simulink model "ultra"  (R2020b)
settings: Solver=FixedStepDiscrete  StartTime=0.0  StopTime=10.0  FixedStep=0.0005  RelTol=1e-3  EnableMultiTasking=on
undefined symbols (not defined in the file): acc_calmax1, acc_calmax2, acc_calmin1, acc_calmin2, akemancanshu, bre, bre_calmax, bre_calmin, ecucoder_acal, I_AN01_5K1, I_AN03_5V, I_AN04_5V, kd, ki, kp, leftmax, O_SW06_HS1A, rightmax, T_add, T_del, tiaoshi, zhiling
libraries: ec5744lib x215, canmsglib x75, simulink x10
(part 4 of 7)

== system ultra/RX/284 286右前/Subsystem2/Subsystem ==
  ID : Inport
  msg : Inport  Port=2
  Enable : EnablePort
  CAN Pack : canmsglib/CAN Pack  Commented=on  CANdbFile=D:\desktop\enable.dbc  MsgList=(none)  MsgName=AMK_ActualValue1  MsgIDType=Standard (11-bit identifier)  MsgIdentifier=643  MsgLength=8  Remote=off  ApplyMinMax=off  BusOutput=off  SignalInfo={'AMK_ActualVelocity','16','16','LE','signed','Standard','0','1','0','0','65535';'AMK_MagnetizingCurrent','48','16','LE','signed','Standard','0','1','0','0','65535';'AMK_TorqueCurrent','32','16','LE','signed','Standard','0','1','0','0','65535';'AMK_bDcOn1','12','1','LE','unsigned','Standard','0','1','0','0','1';'AMK_bDerating1','15','1','LE','unsigned','Standard','0','1','0','0','1';'AMK_bError1','9','1','LE','unsigned','Standard','0','1','0','0','1';'AMK_bInverterOn1','14','1','LE','unsigned','Standard','0','1','0','0','1';'AMK_bQuitDcOn1','11','1','LE','unsigned','Standard','0','1','0','0','1';'AMK_bQuitInverterOn1','13','1','LE','unsigned','Standard','0','1','0','0','1';'AMK_bReserve1','0','8','LE','unsigned','Standard','0','1','0','0','255';'AMK_bSystemReady1','8','1','LE','unsigned','Standard','0','1','0','0','1';'AMK_bWarn1','10','1','LE','unsigned','Standard','0','1','0','0','1'}
      settings: SourceProductBaseCode=ME,XP,VN  DataFormat=CANdb specified signals
  CAN Unpack : canmsglib/CAN Unpack  CANdbFile=D:\desktop\刘科良\HRT23赛季刘科良\CANdbc\enable - youqian.dbc  MsgList=(none)  MsgName=AMK_ActualValue1  MsgIDType=Standard (11-bit identifier)  MsgIdentifier=644  MsgLength=8  SignalInfo={'AMK_ActualVelocity','16','16','LE','signed','Standard','0','1','0','0','65535';'AMK_MagnetizingCurrent','48','16','LE','signed','Standard','0','1','0','0','65535';'AMK_TorqueCurrent','32','16','LE','signed','Standard','0','1','0','0','65535';'AMK_bDcOn1','12','1','LE','unsigned','Standard','0','1','0','0','1';'AMK_bDerating1','15','1','LE','unsigned','Standard','0','1','0','0','1';'AMK_bError1','9','1','LE','unsigned','Standard','0','1','0','0','1';'AMK_bInverterOn1','14','1','LE','unsigned','Standard','0','1','0','0','1';'AMK_bQuitDcOn1','11','1','LE','unsigned','Standard','0','1','0','0','1';'AMK_bQuitInverterOn1','13','1','LE','unsigned','Standard','0','1','0','0','1';'AMK_bReserve1','0','8','LE','unsigned','Standard','0','1','0','0','255';'AMK_bSystemReady1','8','1','LE','unsigned','Standard','0','1','0','0','1';'AMK_bWarn1','10','1','LE','unsigned','Standard','0','1','0','0','1'}  IDPort=off  TimestampPort=off  ErrorPort=off  RemotePort=off  LengthPort=off  StatusPort=off  ApplyMinMax=off
      settings: SourceProductBaseCode=ME,XP,VN  DataFormat=CANdb specified signals
  CANPackMessage : ec5744lib/RapidECU_U4B/04CANCommunication/CANPackMessage  Commented=on  datalength=8  sampletime=-1
      settings: SourceProductName=ECUCoder for MPC5744
  CANUnPackMessage : ec5744lib/RapidECU_U4B/04CANCommunication/CANUnPackMessage  datalength=8  canmessagetype=Standard(11-bit ID)  sampletime=-1
      settings: SourceProductName=ECUCoder for MPC5744
  Data Store Write : DataStoreWrite  DataStoreName=dianji_velcoity_youqian
  Data Store Write1 : DataStoreWrite  DataStoreName=dianji_velcoity_youqian1
  MATLAB Function : MATLAB Function  TreatAsAtomicUnit=on
  wires:
  msg/1 -> CANUnPackMessage/2
  CANUnPackMessage/1 -> CAN Unpack/1
  ID/1 -> CANUnPackMessage/1
  CANPackMessage/1 -> ?
  CAN Pack/1 -> CANPackMessage/1
  CAN Unpack/1 -> Data Store Write1/1, MATLAB Function/1(u)
  MATLAB Function/1(y) -> Data Store Write/1

== system ultra/RX/287 289右后/Subsystem1/Subsystem ==
  ID : Inport
  msg : Inport  Port=2
  Enable : EnablePort
  CAN Pack : canmsglib/CAN Pack  Commented=on  CANdbFile=D:\desktop\enable.dbc  MsgList=(none)  MsgName=AMK_ActualValue1  MsgIDType=Standard (11-bit identifier)  MsgIdentifier=643  MsgLength=8  Remote=off  ApplyMinMax=off  BusOutput=off  SignalInfo={'AMK_ActualVelocity','16','16','LE','signed','Standard','0','1','0','0','65535';'AMK_MagnetizingCurrent','48','16','LE','signed','Standard','0','1','0','0','65535';'AMK_TorqueCurrent','32','16','LE','signed','Standard','0','1','0','0','65535';'AMK_bDcOn1','12','1','LE','unsigned','Standard','0','1','0','0','1';'AMK_bDerating1','15','1','LE','unsigned','Standard','0','1','0','0','1';'AMK_bError1','9','1','LE','unsigned','Standard','0','1','0','0','1';'AMK_bInverterOn1','14','1','LE','unsigned','Standard','0','1','0','0','1';'AMK_bQuitDcOn1','11','1','LE','unsigned','Standard','0','1','0','0','1';'AMK_bQuitInverterOn1','13','1','LE','unsigned','Standard','0','1','0','0','1';'AMK_bReserve1','0','8','LE','unsigned','Standard','0','1','0','0','255';'AMK_bSystemReady1','8','1','LE','unsigned','Standard','0','1','0','0','1';'AMK_bWarn1','10','1','LE','unsigned','Standard','0','1','0','0','1'}
      settings: SourceProductBaseCode=ME,XP,VN  DataFormat=CANdb specified signals
  CAN Unpack : canmsglib/CAN Unpack  CANdbFile=D:\desktop\刘科良\HRT23赛季刘科良\CANdbc\enable - zuohou - 副本.dbc  MsgList=(none)  MsgName=AMK_ActualValue2  MsgIDType=Standard (11-bit identifier)  MsgIdentifier=649  MsgLength=8  SignalInfo={'AMK_ErrorInfo','32','16','LE','unsigned','Standard','0','1','0','0','65535';'AMK_TempIGBT','48','16','LE','signed','Standard','0','1','0','0','65535';'AMK_TempInverter','16','16','LE','signed','Standard','0','1','0','-32768','32767';'AMK_TempMotor','0','16','LE','signed','Standard','0','1','0','0','65535'}  IDPort=off  TimestampPort=off  ErrorPort=off  RemotePort=off  LengthPort=off  StatusPort=off  ApplyMinMax=off
      settings: SourceProductBaseCode=ME,XP,VN  DataFormat=CANdb specified signals
  CANPackMessage : ec5744lib/RapidECU_U4B/04CANCommunication/CANPackMessage  Commented=on  datalength=8  sampletime=-1
      settings: SourceProductName=ECUCoder for MPC5744
  CANUnPackMessage : ec5744lib/RapidECU_U4B/04CANCommunication/CANUnPackMessage  datalength=8  canmessagetype=Standard(11-bit ID)  sampletime=-1
      settings: SourceProductName=ECUCoder for MPC5744
  wires:
  msg/1 -> CANUnPackMessage/2
  CANUnPackMessage/1 -> CAN Unpack/1
  ID/1 -> CANUnPackMessage/1
  CANPackMessage/1 -> ?
  CAN Pack/1 -> CANPackMessage/1

== system ultra/RX/287 289右后/Subsystem2/Subsystem ==
  ID : Inport
  msg : Inport  Port=2
  Enable : EnablePort
  CAN Pack : canmsglib/CAN Pack  Commented=on  CANdbFile=D:\desktop\enable.dbc  MsgList=(none)  MsgName=AMK_ActualValue1  MsgIDType=Standard (11-bit identifier)  MsgIdentifier=643  MsgLength=8  Remote=off  ApplyMinMax=off  BusOutput=off  SignalInfo={'AMK_ActualVelocity','16','16','LE','signed','Standard','0','1','0','0','65535';'AMK_MagnetizingCurrent','48','16','LE','signed','Standard','0','1','0','0','65535';'AMK_TorqueCurrent','32','16','LE','signed','Standard','0','1','0','0','65535';'AMK_bDcOn1','12','1','LE','unsigned','Standard','0','1','0','0','1';'AMK_bDerating1','15','1','LE','unsigned','Standard','0','1','0','0','1';'AMK_bError1','9','1','LE','unsigned','Standard','0','1','0','0','1';'AMK_bInverterOn1','14','1','LE','unsigned','Standard','0','1','0','0','1';'AMK_bQuitDcOn1','11','1','LE','unsigned','Standard','0','1','0','0','1';'AMK_bQuitInverterOn1','13','1','LE','unsigned','Standard','0','1','0','0','1';'AMK_bReserve1','0','8','LE','unsigned','Standard','0','1','0','0','255';'AMK_bSystemReady1','8','1','LE','unsigned','Standard','0','1','0','0','1';'AMK_bWarn1','10','1','LE','unsigned','Standard','0','1','0','0','1'}
      settings: SourceProductBaseCode=ME,XP,VN  DataFormat=CANdb specified signals
  CAN Unpack : canmsglib/CAN Unpack  CANdbFile=C:\Users\Liu keliang\Desktop\HRT2023\HRT23赛季刘科良\CANdbc\enable - zuohou - 副本.dbc  MsgList=(none)  MsgName=AMK_ActualValue1  MsgIDType=Standard (11-bit identifier)  MsgIdentifier=647  MsgLength=8  SignalInfo={'AMK_ActualVelocity','16','16','LE','signed','Standard','0','1','0','0','65535';'AMK_MagnetizingCurrent','48','16','LE','signed','Standard','0','1','0','0','65535';'AMK_TorqueCurrent','32','16','LE','signed','Standard','0','1','0','0','65535';'AMK_bDcOn1','12','1','LE','unsigned','Standard','0','1','0','0','1';'AMK_bDerating1','15','1','LE','unsigned','Standard','0','1','0','0','1';'AMK_bError1','9','1','LE','unsigned','Standard','0','1','0','0','1';'AMK_bInverterOn1','14','1','LE','unsigned','Standard','0','1','0','0','1';'AMK_bQuitDcOn1','11','1','LE','unsigned','Standard','0','1','0','0','1';'AMK_bQuitInverterOn1','13','1','LE','unsigned','Standard','0','1','0','0','1';'AMK_bReserve1','0','8','LE','unsigned','Standard','0','1','0','0','255';'AMK_bSystemReady1','8','1','LE','unsigned','Standard','0','1','0','0','1';'AMK_bWarn1','10','1','LE','unsigned','Standard','0','1','0','0','1'}  IDPort=off  TimestampPort=off  ErrorPort=off  RemotePort=off  LengthPort=off  StatusPort=off  ApplyMinMax=off
      settings: SourceProductBaseCode=ME,XP,VN  DataFormat=CANdb specified signals
  CANPackMessage : ec5744lib/RapidECU_U4B/04CANCommunication/CANPackMessage  Commented=on  datalength=8  sampletime=-1
      settings: SourceProductName=ECUCoder for MPC5744
  CANUnPackMessage : ec5744lib/RapidECU_U4B/04CANCommunication/CANUnPackMessage  datalength=8  canmessagetype=Standard(11-bit ID)  sampletime=-1
      settings: SourceProductName=ECUCoder for MPC5744
  Data Store Write : DataStoreWrite  DataStoreName=dianji_velcoity_zuohou
  MATLAB Function : MATLAB Function  TreatAsAtomicUnit=on
  wires:
  msg/1 -> CANUnPackMessage/2
  CANUnPackMessage/1 -> CAN Unpack/1
  ID/1 -> CANUnPackMessage/1
  CANPackMessage/1 -> ?
  CAN Pack/1 -> CANPackMessage/1
  CAN Unpack/1 -> MATLAB Function/1(u)
  MATLAB Function/1(y) -> Data Store Write/1

== system ultra/RX/287 289右后/Subsystem3/Subsystem ==
  ID : Inport
  msg : Inport  Port=2
  Enable : EnablePort
  CAN Pack : canmsglib/CAN Pack  Commented=on  CANdbFile=D:\desktop\enable.dbc  MsgList=(none)  MsgName=AMK_ActualValue1  MsgIDType=Standard (11-bit identifier)  MsgIdentifier=643  MsgLength=8  Remote=off  ApplyMinMax=off  BusOutput=off  SignalInfo={'AMK_ActualVelocity','16','16','LE','signed','Standard','0','1','0','0','65535';'AMK_MagnetizingCurrent','48','16','LE','signed','Standard','0','1','0','0','65535';'AMK_TorqueCurrent','32','16','LE','signed','Standard','0','1','0','0','65535';'AMK_bDcOn1','12','1','LE','unsigned','Standard','0','1','0','0','1';'AMK_bDerating1','15','1','LE','unsigned','Standard','0','1','0','0','1';'AMK_bError1','9','1','LE','unsigned','Standard','0','1','0','0','1';'AMK_bInverterOn1','14','1','LE','unsigned','Standard','0','1','0','0','1';'AMK_bQuitDcOn1','11','1','LE','unsigned','Standard','0','1','0','0','1';'AMK_bQuitInverterOn1','13','1','LE','unsigned','Standard','0','1','0','0','1';'AMK_bReserve1','0','8','LE','unsigned','Standard','0','1','0','0','255';'AMK_bSystemReady1','8','1','LE','unsigned','Standard','0','1','0','0','1';'AMK_bWarn1','10','1','LE','unsigned','Standard','0','1','0','0','1'}
      settings: SourceProductBaseCode=ME,XP,VN  DataFormat=CANdb specified signals
  CAN Unpack : canmsglib/CAN Unpack  CANdbFile=C:\Users\Liu keliang\Desktop\HRT2023\HRT23赛季刘科良\CANdbc\enable - 副本.dbc  MsgList=AMK_ActualValue1  MsgName=AMK_ActualValue1  MsgIDType=Standard (11-bit identifier)  MsgIdentifier=647  MsgLength=8  SignalInfo={'AMK_ActualVelocity','16','16','LE','signed','Standard','0','1','0','0','65535';'AMK_MagnetizingCurrent','48','16','LE','signed','Standard','0','1','0','0','65535';'AMK_TorqueCurrent','32','16','LE','signed','Standard','0','1','0','0','65535';'AMK_bDcOn1','12','1','LE','unsigned','Standard','0','1','0','0','1';'AMK_bDerating1','15','1','LE','unsigned','Standard','0','1','0','0','1';'AMK_bError1','9','1','LE','unsigned','Standard','0','1','0','0','1';'AMK_bInverterOn1','14','1','LE','unsigned','Standard','0','1','0','0','1';'AMK_bQuitDcOn1','11','1','LE','unsigned','Standard','0','1','0','0','1';'AMK_bQuitInverterOn1','13','1','LE','unsigned','Standard','0','1','0','0','1';'AMK_bReserve1','0','8','LE','unsigned','Standard','0','1','0','0','255';'AMK_bSystemReady1','8','1','LE','unsigned','Standard','0','1','0','0','1';'AMK_bWarn1','10','1','LE','unsigned','Standard','0','1','0','0','1'}  IDPort=off  TimestampPort=off  ErrorPort=off  RemotePort=off  LengthPort=off  StatusPort=off  ApplyMinMax=off
      settings: SourceProductBaseCode=ME,XP,VN  DataFormat=CANdb specified signals
  CANPackMessage : ec5744lib/RapidECU_U4B/04CANCommunication/CANPackMessage  Commented=on  datalength=8  sampletime=-1
      settings: SourceProductName=ECUCoder for MPC5744
  CANUnPackMessage : ec5744lib/RapidECU_U4B/04CANCommunication/CANUnPackMessage  datalength=8  canmessagetype=Standard(11-bit ID)  sampletime=-1
      settings: SourceProductName=ECUCoder for MPC5744
  Data Store Write : DataStoreWrite  DataStoreName=dianji_velcoity_youhou
  Data Store Write1 : DataStoreWrite  DataStoreName=dianji_velcoity_youhou1
  MATLAB Function : MATLAB Function  TreatAsAtomicUnit=on
  wires:
  msg/1 -> CANUnPackMessage/2
  CANUnPackMessage/1 -> CAN Unpack/1
  ID/1 -> CANUnPackMessage/1
  CANPackMessage/1 -> ?
  CAN Pack/1 -> CANPackMessage/1
  MATLAB Function/1(y) -> Data Store Write/1
  CAN Unpack/1 -> Data Store Write1/1, MATLAB Function/1(u)

== system ultra/RX/288 290左后/Subsystem1/Subsystem ==
  ID : Inport
  msg : Inport  Port=2
  Enable : EnablePort
  CAN Pack : canmsglib/CAN Pack  Commented=on  CANdbFile=D:\desktop\enable.dbc  MsgList=(none)  MsgName=AMK_ActualValue1  MsgIDType=Standard (11-bit identifier)  MsgIdentifier=643  MsgLength=8  Remote=off  ApplyMinMax=off  BusOutput=off  SignalInfo={'AMK_ActualVelocity','16','16','LE','signed','Standard','0','1','0','0','65535';'AMK_MagnetizingCurrent','48','16','LE','signed','Standard','0','1','0','0','65535';'AMK_TorqueCurrent','32','16','LE','signed','Standard','0','1','0','0','65535';'AMK_bDcOn1','12','1','LE','unsigned','Standard','0','1','0','0','1';'AMK_bDerating1','15','1','LE','unsigned','Standard','0','1','0','0','1';'AMK_bError1','9','1','LE','unsigned','Standard','0','1','0','0','1';'AMK_bInverterOn1','14','1','LE','unsigned','Standard','0','1','0','0','1';'AMK_bQuitDcOn1','11','1','LE','unsigned','Standard','0','1','0','0','1';'AMK_bQuitInverterOn1','13','1','LE','unsigned','Standard','0','1','0','0','1';'AMK_bReserve1','0','8','LE','unsigned','Standard','0','1','0','0','255';'AMK_bSystemReady1','8','1','LE','unsigned','Standard','0','1','0','0','1';'AMK_bWarn1','10','1','LE','unsigned','Standard','0','1','0','0','1'}
      settings: SourceProductBaseCode=ME,XP,VN  DataFormat=CANdb specified signals
  CAN Unpack : canmsglib/CAN Unpack  CANdbFile=D:\desktop\刘科良\HRT23赛季刘科良\CANdbc\enable - youhou -.dbc  MsgList=(none)  MsgName=AMK_ActualValue2  MsgIDType=Standard (11-bit identifier)  MsgIdentifier=656  MsgLength=8  SignalInfo={'AMK_ErrorInfo','32','16','LE','unsigned','Standard','0','1','0','0','65535';'AMK_TempIGBT','48','16','LE','signed','Standard','0','1','0','0','65535';'AMK_TempInverter','16','16','LE','signed','Standard','0','1','0','-32768','32767';'AMK_TempMotor','0','16','LE','signed','Standard','0','1','0','0','65535'}  IDPort=off  TimestampPort=off  ErrorPort=off  RemotePort=off  LengthPort=off  StatusPort=off  ApplyMinMax=off
      settings: SourceProductBaseCode=ME,XP,VN  DataFormat=CANdb specified signals
  CANPackMessage : ec5744lib/RapidECU_U4B/04CANCommunication/CANPackMessage  Commented=on  datalength=8  sampletime=-1
      settings: SourceProductName=ECUCoder for MPC5744
  CANUnPackMessage : ec5744lib/RapidECU_U4B/04CANCommunication/CANUnPackMessage  datalength=8  canmessagetype=Standard(11-bit ID)  sampletime=-1
      settings: SourceProductName=ECUCoder for MPC5744
  wires:
  msg/1 -> CANUnPackMessage/2
  CANUnPackMessage/1 -> CAN Unpack/1
  ID/1 -> CANUnPackMessage/1
  CANPackMessage/1 -> ?
  CAN Pack/1 -> CANPackMessage/1

== system ultra/RX/288 290左后/Subsystem2/Subsystem ==
  ID : Inport
  msg : Inport  Port=2
  Enable : EnablePort
  CAN Pack : canmsglib/CAN Pack  Commented=on  CANdbFile=D:\desktop\enable.dbc  MsgList=(none)  MsgName=AMK_ActualValue1  MsgIDType=Standard (11-bit identifier)  MsgIdentifier=643  MsgLength=8  Remote=off  ApplyMinMax=off  BusOutput=off  SignalInfo={'AMK_ActualVelocity','16','16','LE','signed','Standard','0','1','0','0','65535';'AMK_MagnetizingCurrent','48','16','LE','signed','Standard','0','1','0','0','65535';'AMK_TorqueCurrent','32','16','LE','signed','Standard','0','1','0','0','65535';'AMK_bDcOn1','12','1','LE','unsigned','Standard','0','1','0','0','1';'AMK_bDerating1','15','1','LE','unsigned','Standard','0','1','0','0','1';'AMK_bError1','9','1','LE','unsigned','Standard','0','1','0','0','1';'AMK_bInverterOn1','14','1','LE','unsigned','Standard','0','1','0','0','1';'AMK_bQuitDcOn1','11','1','LE','unsigned','Standard','0','1','0','0','1';'AMK_bQuitInverterOn1','13','1','LE','unsigned','Standard','0','1','0','0','1';'AMK_bReserve1','0','8','LE','unsigned','Standard','0','1','0','0','255';'AMK_bSystemReady1','8','1','LE','unsigned','Standard','0','1','0','0','1';'AMK_bWarn1','10','1','LE','unsigned','Standard','0','1','0','0','1'}
      settings: SourceProductBaseCode=ME,XP,VN  DataFormat=CANdb specified signals
  CAN Unpack : canmsglib/CAN Unpack  CANdbFile=D:\desktop\刘科良\HRT23赛季刘科良\CANdbc\enable - youhou -.dbc  MsgList=(none)  MsgName=AMK_ActualValue1  MsgIDType=Standard (11-bit identifier)  MsgIdentifier=648  MsgLength=8  SignalInfo={'AMK_ActualVelocity','16','16','LE','signed','Standard','0','1','0','0','65535';'AMK_MagnetizingCurrent','48','16','LE','signed','Standard','0','1','0','0','65535';'AMK_TorqueCurrent','32','16','LE','signed','Standard','0','1','0','0','65535';'AMK_bDcOn1','12','1','LE','unsigned','Standard','0','1','0','0','1';'AMK_bDerating1','15','1','LE','unsigned','Standard','0','1','0','0','1';'AMK_bError1','9','1','LE','unsigned','Standard','0','1','0','0','1';'AMK_bInverterOn1','14','1','LE','unsigned','Standard','0','1','0','0','1';'AMK_bQuitDcOn1','11','1','LE','unsigned','Standard','0','1','0','0','1';'AMK_bQuitInverterOn1','13','1','LE','unsigned','Standard','0','1','0','0','1';'AMK_bReserve1','0','8','LE','unsigned','Standard','0','1','0','0','255';'AMK_bSystemReady1','8','1','LE','unsigned','Standard','0','1','0','0','1';'AMK_bWarn1','10','1','LE','unsigned','Standard','0','1','0','0','1'}  IDPort=off  TimestampPort=off  ErrorPort=off  RemotePort=off  LengthPort=off  StatusPort=off  ApplyMinMax=off
      settings: SourceProductBaseCode=ME,XP,VN  DataFormat=CANdb specified signals
  CANPackMessage : ec5744lib/RapidECU_U4B/04CANCommunication/CANPackMessage  Commented=on  datalength=8  sampletime=-1
      settings: SourceProductName=ECUCoder for MPC5744
  CANUnPackMessage : ec5744lib/RapidECU_U4B/04CANCommunication/CANUnPackMessage  datalength=8  canmessagetype=Standard(11-bit ID)  sampletime=-1
      settings: SourceProductName=ECUCoder for MPC5744
  Data Store Write : DataStoreWrite  DataStoreName=dianji_velcoity_zuohou
  Data Store Write1 : DataStoreWrite  DataStoreName=dianji_velcoity_zuohou1
  MATLAB Function : MATLAB Function  TreatAsAtomicUnit=on
  wires:
  msg/1 -> CANUnPackMessage/2
  CANUnPackMessage/1 -> CAN Unpack/1
  ID/1 -> CANUnPackMessage/1
  CANPackMessage/1 -> ?
  CAN Pack/1 -> CANPackMessage/1
  CAN Unpack/1 -> Data Store Write1/1, MATLAB Function/1(u)
  MATLAB Function/1(y) -> Data Store Write/1

== system ultra/RX/ebs/Subsystem3/Subsystem ==
  ID : Inport
  msg : Inport  Port=2
  Enable : EnablePort
  CAN Pack : canmsglib/CAN Pack  Commented=on  CANdbFile=C:\Users\Liu keliang\Desktop\HRT2023\HRT23赛季刘科良\CANdbc\workstation.dbc  MsgList=(none)  MsgName=workstation  MsgIDType=Standard (11-bit identifier)  MsgIdentifier=32  MsgLength=5  Remote=off  ApplyMinMax=off  BusOutput=off  SignalInfo={'V','8','8','LE','unsigned','Standard','0','1','0','0','255';'V_Copy_1','16','8','LE','unsigned','Standard','0','1','0','0','255';'controlstart','4','1','LE','unsigned','Standard','0','1','0','-Inf','Inf';'status','0','4','LE','unsigned','Standard','0','1','0','0','15';'steering','24','8','LE','signed','Standard','0','1','0','-128','127';'steering_Copy_1','32','8','LE','signed','Standard','0','1','0','-128','127';'vfeedbackk','40','8','LE','unsigned','Standard','0','1','0','-Inf','Inf'}
      settings: SourceProductBaseCode=ME,XP,VN  DataFormat=CANdb specified signals
  CAN Unpack : canmsglib/CAN Unpack  CANdbFile=C:\Users\Liu keliang\Desktop\HRT2023\HRT23赛季刘科良\CANdbc\ebs.dbc  MsgList=New_Message_1  MsgName=New_Message_1  MsgIDType=Standard (11-bit identifier)  MsgIdentifier=1026  MsgLength=8  SignalInfo={'youhou','48','16','LE','unsigned','Standard','0','1','0','-Inf','Inf';'youqian','16','16','LE','unsigned','Standard','0','1','0','-Inf','Inf';'zuohou','32','16','LE','unsigned','Standard','0','1','0','-Inf','Inf';'zuoqian','0','16','LE','unsigned','Standard','0','1','0','-Inf','Inf'}  IDPort=off  TimestampPort=off  ErrorPort=off  RemotePort=off  LengthPort=off  StatusPort=off  ApplyMinMax=off
      settings: SourceProductBaseCode=ME,XP,VN  DataFormat=CANdb specified signals
  CANPackMessage : ec5744lib/RapidECU_U4B/04CANCommunication/CANPackMessage  Commented=on  datalength=8  sampletime=-1
      settings: SourceProductName=ECUCoder for MPC5744
  CANUnPackMessage : ec5744lib/RapidECU_U4B/04CANCommunication/CANUnPackMessage  datalength=8  canmessagetype=Standard(11-bit ID)  sampletime=-1
      settings: SourceProductName=ECUCoder for MPC5744
  Data Store Write : DataStoreWrite  DataStoreName=oilyouhou
  Data Store Write1 : DataStoreWrite  DataStoreName=oilyouqian
  Data Store Write2 : DataStoreWrite  DataStoreName=oilzuohou
  Data Store Write3 : DataStoreWrite  DataStoreName=oilzuoqian
  wires:
  msg/1 -> CANUnPackMessage/2
  CANUnPackMessage/1 -> CAN Unpack/1
  ID/1 -> CANUnPackMessage/1
  CANPackMessage/1 -> ?
  CAN Pack/1 -> CANPackMessage/1
  CAN Unpack/2 -> Data Store Write1/1
  CAN Unpack/1 -> Data Store Write/1
  CAN Unpack/3 -> Data Store Write2/1
  CAN Unpack/4 -> Data Store Write3/1

== system ultra/RX/lcu——receive/Subsystem1/Subsystem ==
  ID : Inport
  msg : Inport  Port=2
  Enable : EnablePort
  CAN Pack : canmsglib/CAN Pack  Commented=on  CANdbFile=C:\Users\Liu keliang\Desktop\HRT2023\HRT23赛季刘科良\CANdbc\enzbled.dbc  MsgList=(none)  MsgName=ecu156  MsgIDType=Standard (11-bit identifier)  MsgIdentifier=342  MsgLength=8  Remote=off  ApplyMinMax=off  BusOutput=off  SignalInfo={'ASMS','3','1','LE','unsigned','Standard','0','1','0','-Inf','Inf';'enable','32','8','LE','unsigned','Standard','0','1','0','0','255';'error','16','8','LE','unsigned','Standard','0','1','0','0','255';'match_model','8','4','LE','unsigned','Standard','0','1','0','0','15';'matchmodel_shucai','24','3','LE','unsigned','Standard','0','1','0','0','6';'model_confirm','27','1','LE','unsigned','Standard','0','1','0','0','1';'res','40','3','LE','unsigned','Standard','0','1','0','-Inf','Inf';'ststus','0','3','LE','unsigned','Standard','0','1','0','0','7'}
      settings: SourceProductBaseCode=ME,XP,VN  DataFormat=CANdb specified signals
  CAN Unpack : canmsglib/CAN Unpack  CANdbFile=C:\Users\Liu keliang\Desktop\HRT2023\HRT23赛季刘科良\CANdbc\enzbled.dbc  MsgList=ecu156  MsgName=ecu156  MsgIDType=Standard (11-bit identifier)  MsgIdentifier=342  MsgLength=8  SignalInfo={'ASMS','3','1','LE','unsigned','Standard','0','1','0','-Inf','Inf';'enable','32','8','LE','unsigned','Standard','0','1','0','0','255';'error','16','8','LE','unsigned','Standard','0','1','0','0','255';'match_model','8','4','LE','unsigned','Standard','0','1','0','0','15';'matchmodel_shucai','24','3','LE','unsigned','Standard','0','1','0','0','6';'model_confirm','27','1','LE','unsigned','Standard','0','1','0','0','1';'res','40','3','LE','unsigned','Standard','0','1','0','-Inf','Inf';'ststus','0','3','LE','unsigned','Standard','0','1','0','0','7'}  IDPort=off  TimestampPort=off  ErrorPort=off  RemotePort=off  LengthPort=off  StatusPort=off  ApplyMinMax=off
      settings: SourceProductBaseCode=ME,XP,VN  DataFormat=CANdb specified signals
  CANPackMessage : ec5744lib/RapidECU_U4B/04CANCommunication/CANPackMessage  Commented=on  datalength=8  sampletime=-1
      settings: SourceProductName=ECUCoder for MPC5744
  CANUnPackMessage : ec5744lib/RapidECU_U4B/04CANCommunication/CANUnPackMessage  datalength=8  canmessagetype=Standard(11-bit ID)  sampletime=-1
      settings: SourceProductName=ECUCoder for MPC5744
  Data Store Read : DataStoreRead  DataStoreName=status
  Data Store Write : DataStoreWrite  DataStoreName=match_model
  Data Store Write1 : DataStoreWrite  DataStoreName=status
  Data Store Write2 : DataStoreWrite  DataStoreName=nengpao
  MATLAB Function : MATLAB Function  Commented=on  TreatAsAtomicUnit=on
  MATLAB Function1 : MATLAB Function  TreatAsAtomicUnit=on
  MATLAB Function2 : MATLAB Function  TreatAsAtomicUnit=on
  MeaModule8 : ec5744lib/RapidECU_U4B/07Calibration/MeaModule  signal=enable
      settings: SourceProductName=ECUCoder for MPC5744
  缓停 : DataStoreWrite  DataStoreName=huanting
  Out1 : Outport
  CAN_msg_enable : Outport  Port=2
  wires:
  msg/1 -> CANUnPackMessage/2
  CANUnPackMessage/1 -> CAN Unpack/1
  ID/1 -> CANUnPackMessage/1
  CANPackMessage/1 -> Out1/1
  CAN Pack/1 -> CANPackMessage/1
  CAN Unpack/3 -> CAN Pack/3
  CAN Unpack/4 -> Data Store Write/1, CAN Pack/4
  CAN Unpack/5 -> CAN Pack/5
  CAN Unpack/6 -> CAN Pack/6
  MeaModule8/1 -> CAN_msg_enable/1
  CAN Unpack/1 -> CAN Pack/1
  CAN Unpack/2 -> MeaModule8/1, CAN Pack/2
  MATLAB Function1/1(y) -> 缓停/1
  Data Store Read/1 -> MATLAB Function2/1(u)
  MATLAB Function2/1(y) -> Data Store Write2/1
  CAN Unpack/8 -> Data Store Write1/1, MATLAB Function1/1(u)

== system ultra/RX/工作站/Subsystem1/Subsystem1 ==
  ID : Inport
  msg : Inport  Port=2
  Enable : EnablePort
  Subsystem : Subsystem
  wires:
  ID/1 -> Subsystem/1(ID)
  msg/1 -> Subsystem/2(msg)

== system ultra/RX/工作站/Subsystem3/Subsystem ==
  ID : Inport
  msg : Inport  Port=2
  Enable : EnablePort
  Add : Sum
  Add1 : Sum
  CAN Pack : canmsglib/CAN Pack  Commented=on  CANdbFile=C:\Users\Liu keliang\Desktop\HRT2023\HRT23赛季刘科良\CANdbc\workstation.dbc  MsgList=(none)  MsgName=workstation  MsgIDType=Standard (11-bit identifier)  MsgIdentifier=32  MsgLength=5  Remote=off  ApplyMinMax=off  BusOutput=off  SignalInfo={'V','8','8','LE','unsigned','Standard','0','1','0','0','255';'V_Copy_1','16','8','LE','unsigned','Standard','0','1','0','0','255';'controlstart','4','1','LE','unsigned','Standard','0','1','0','-Inf','Inf';'status','0','4','LE','unsigned','Standard','0','1','0','0','15';'steering','24','8','LE','signed','Standard','0','1','0','-128','127';'steering_Copy_1','32','8','LE','signed','Standard','0','1','0','-128','127';'vfeedbackk','40','8','LE','unsigned','Standard','0','1','0','-Inf','Inf'}
      settings: SourceProductBaseCode=ME,XP,VN  DataFormat=CANdb specified signals
  CAN Unpack : canmsglib/CAN Unpack  CANdbFile=C:\Users\Liu keliang\Desktop\HRT2023\HRT23赛季刘科良\CANdbc\workstation.dbc  MsgList=workstation  MsgName=workstation  MsgIDType=Standard (11-bit identifier)  MsgIdentifier=32  MsgLength=6  SignalInfo={'V','8','8','LE','unsigned','Standard','0','1','0','0','255';'V_Copy_1','16','8','LE','unsigned','Standard','0','1','0','0','255';'jiting','40','4','LE','unsigned','Standard','0','1','0','0','8';'status','0','4','LE','unsigned','Standard','0','1','0','0','15';'steering','24','8','LE','signed','Standard','0','1','0','-128','127';'steering_Copy_1','32','8','LE','signed','Standard','0','1','0','-128','127'}  IDPort=off  TimestampPort=off  ErrorPort=off  RemotePort=off  LengthPort=off  StatusPort=off  ApplyMinMax=off
      settings: SourceProductBaseCode=ME,XP,VN  DataFormat=CANdb specified signals
  CANPackMessage : ec5744lib/RapidECU_U4B/04CANCommunication/CANPackMessage  Commented=on  datalength=8  sampletime=-1
      settings: SourceProductName=ECUCoder for MPC5744
  CANUnPackMessage : ec5744lib/RapidECU_U4B/04CANCommunication/CANUnPackMessage  datalength=6  canmessagetype=Standard(11-bit ID)  sampletime=-1
      settings: SourceProductName=ECUCoder for MPC5744
  Data Store Read1 : DataStoreRead  DataStoreName=nengpao
  Data Store Read3 : DataStoreRead  DataStoreName=match_model
  Data Store Write : DataStoreWrite  DataStoreName=V_workstation
  Data Store Write1 : DataStoreWrite  DataStoreName=workstation_status
  Data Store Write2 : DataStoreWrite  DataStoreName=workstation_steering
  Data Store Write3 : DataStoreWrite  DataStoreName=jiting
  MATLAB Function : MATLAB Function  TreatAsAtomicUnit=on
  MATLAB Function1 : MATLAB Function  TreatAsAtomicUnit=on
  MATLAB Function2 : MATLAB Function  TreatAsAtomicUnit=on
  MATLAB Function3 : MATLAB Function  TreatAsAtomicUnit=on
  MATLAB Function4 : MATLAB Function  TreatAsAtomicUnit=on
  Subsystem : Subsystem
  wires:
  msg/1 -> CANUnPackMessage/2
  CANUnPackMessage/1 -> CAN Unpack/1
  ID/1 -> CANUnPackMessage/1
  CANPackMessage/1 -> ?
  CAN Pack/1 -> CANPackMessage/1
  CAN Unpack/1 -> MATLAB Function/1(u)
  Add1/1 -> Data Store Write2/1
  MATLAB Function/1(y) -> Add/1
  MATLAB Function2/1(y) -> Add/2
  MATLAB Function3/1(y) -> Add1/2
  MATLAB Function1/1(y) -> Add1/1
  MATLAB Function4/1(y) -> Data Store Write/1
  Data Store Read1/1 -> MATLAB Function4/2(nengbunengpao)
  Add/1 -> MATLAB Function4/1(u)
  CAN Unpack/4 -> Data Store Write1/1
  CAN Unpack/5 -> MATLAB Function1/1(u)
  CAN Unpack/6 -> MATLAB Function3/1(u)
  Data Store Read3/1 -> MATLAB Function4/3(model)
  CAN Unpack/3 -> Data Store Write3/1
  CAN Unpack/2 -> MATLAB Function2/1(u)
  Subsystem/1(Out1) -> MATLAB Function3/2(CANOK_20), MATLAB Function1/2(CANOK_20), MATLAB Function2/2(CANOK_20), MATLAB Function/2(CANOK_20)

== system ultra/RX/惯导/Subsystem1/Subsystem ==
  ID : Inport
  msg : Inport  Port=2
  Enable : EnablePort
  CAN Pack : canmsglib/CAN Pack  Commented=on  CANdbFile=D:\desktop\enable.dbc  MsgList=(none)  MsgName=AMK_ActualValue1  MsgIDType=Standard (11-bit identifier)  MsgIdentifier=643  MsgLength=8  Remote=off  ApplyMinMax=off  BusOutput=off  SignalInfo={'AMK_ActualVelocity','16','16','LE','signed','Standard','0','1','0','0','65535';'AMK_MagnetizingCurrent','48','16','LE','signed','Standard','0','1','0','0','65535';'AMK_TorqueCurrent','32','16','LE','signed','Standard','0','1','0','0','65535';'AMK_bDcOn1','12','1','LE','unsigned','Standard','0','1','0','0','1';'AMK_bDerating1','15','1','LE','unsigned','Standard','0','1','0','0','1';'AMK_bError1','9','1','LE','unsigned','Standard','0','1','0','0','1';'AMK_bInverterOn1','14','1','LE','unsigned','Standard','0','1','0','0','1';'AMK_bQuitDcOn1','11','1','LE','unsigned','Standard','0','1','0','0','1';'AMK_bQuitInverterOn1','13','1','LE','unsigned','Standard','0','1','0','0','1';'AMK_bReserve1','0','8','LE','unsigned','Standard','0','1','0','0','255';'AMK_bSystemReady1','8','1','LE','unsigned','Standard','0','1','0','0','1';'AMK_bWarn1','10','1','LE','unsigned','Standard','0','1','0','0','1'}
      settings: SourceProductBaseCode=ME,XP,VN  DataFormat=CANdb specified signals
  CAN Unpack : canmsglib/CAN Unpack  CANdbFile=C:\Users\Liu keliang\Desktop\HRT2023\HRT23赛季刘科良\CANdbc\homework1.dbc  MsgList=INS_HeadingPitchRoll  MsgName=INS_HeadingPitchRoll  MsgIDType=Standard (11-bit identifier)  MsgIdentifier=1282  MsgLength=7  SignalInfo={'INS_HeadingAngle','48','16','BE','unsigned','Standard','0','0.010986','-360','-360','360';'INS_PitchAngle','16','16','BE','unsigned','Standard','0','0.010986','-360','-360','360';'INS_RollAngle','32','16','BE','unsigned','Standard','0','0.010986','-360','-360','360'}  IDPort=off  TimestampPort=off  ErrorPort=off  RemotePort=off  LengthPort=off  StatusPort=off  ApplyMinMax=off
      settings: SourceProductBaseCode=ME,XP,VN  DataFormat=CANdb specified signals
  CANPackMessage : ec5744lib/RapidECU_U4B/04CANCommunication/CANPackMessage  Commented=on  datalength=8  sampletime=-1
      settings: SourceProductName=ECUCoder for MPC5744
  CANUnPackMessage : ec5744lib/RapidECU_U4B/04CANCommunication/CANUnPackMessage  datalength=7  canmessagetype=Standard(11-bit ID)  sampletime=-1
      settings: SourceProductName=ECUCoder for MPC5744
  Data Store Write : DataStoreWrite  DataStoreName=HEADING_ANGLE
  wires:
  msg/1 -> CANUnPackMessage/2
  CANUnPackMessage/1 -> CAN Unpack/1
  ID/1 -> CANUnPackMessage/1
  CANPackMessage/1 -> ?
  CAN Pack/1 -> CANPackMessage/1
  CAN Unpack/1 -> Data Store Write/1

== system ultra/RX/惯导/Subsystem2/Subsystem ==
  ID : Inport
  msg : Inport  Port=2
  Enable : EnablePort
  CAN Pack : canmsglib/CAN Pack  Commented=on  CANdbFile=D:\desktop\enable.dbc  MsgList=(none)  MsgName=AMK_ActualValue1  MsgIDType=Standard (11-bit identifier)  MsgIdentifier=643  MsgLength=8  Remote=off  ApplyMinMax=off  BusOutput=off  SignalInfo={'AMK_ActualVelocity','16','16','LE','signed','Standard','0','1','0','0','65535';'AMK_MagnetizingCurrent','48','16','LE','signed','Standard','0','1','0','0','65535';'AMK_TorqueCurrent','32','16','LE','signed','Standard','0','1','0','0','65535';'AMK_bDcOn1','12','1','LE','unsigned','Standard','0','1','0','0','1';'AMK_bDerating1','15','1','LE','unsigned','Standard','0','1','0','0','1';'AMK_bError1','9','1','LE','unsigned','Standard','0','1','0','0','1';'AMK_bInverterOn1','14','1','LE','unsigned','Standard','0','1','0','0','1';'AMK_bQuitDcOn1','11','1','LE','unsigned','Standard','0','1','0','0','1';'AMK_bQuitInverterOn1','13','1','LE','unsigned','Standard','0','1','0','0','1';'AMK_bReserve1','0','8','LE','unsigned','Standard','0','1','0','0','255';'AMK_bSystemReady1','8','1','LE','unsigned','Standard','0','1','0','0','1';'AMK_bWarn1','10','1','LE','unsigned','Standard','0','1','0','0','1'}
      settings: SourceProductBaseCode=ME,XP,VN  DataFormat=CANdb specified signals
  CAN Unpack : canmsglib/CAN Unpack  CANdbFile=C:\Users\Liu keliang\Desktop\HRT2023\HRT23赛季刘科良\CANdbc\homework1.dbc  MsgList=INS_Acc  MsgName=INS_Acc  MsgIDType=Standard (11-bit identifier)  MsgIdentifier=1280  MsgLength=7  SignalInfo={'ACC_X','16','16','BE','unsigned','Standard','0','0.000122','-4','-4','4';'ACC_Y','32','16','BE','unsigned','Standard','0','0.000122','-4','-4','4';'ACC_Z','48','16','BE','unsigned','Standard','0','0.000122','-4','-4','4'}  IDPort=off  TimestampPort=off  ErrorPort=off  RemotePort=off  LengthPort=off  StatusPort=off  ApplyMinMax=off
      settings: SourceProductBaseCode=ME,XP,VN  DataFormat=CANdb specified signals
  CANPackMessage : ec5744lib/RapidECU_U4B/04CANCommunication/CANPackMessage  Commented=on  datalength=8  sampletime=-1
      settings: SourceProductName=ECUCoder for MPC5744
  CANUnPackMessage : ec5744lib/RapidECU_U4B/04CANCommunication/CANUnPackMessage  datalength=7  canmessagetype=Standard(11-bit ID)  sampletime=-1
      settings: SourceProductName=ECUCoder for MPC5744
  Data Store Write : DataStoreWrite  DataStoreName=ACC_X
  Data Store Write1 : DataStoreWrite  DataStoreName=ACC_Y
  Data Store Write2 : DataStoreWrite  DataStoreName=ACC_Z
  wires:
  msg/1 -> CANUnPackMessage/2
  CANUnPackMessage/1 -> CAN Unpack/1
  ID/1 -> CANUnPackMessage/1
  CANPackMessage/1 -> ?
  CAN Pack/1 -> CANPackMessage/1
  CAN Unpack/1 -> Data Store Write/1
  CAN Unpack/2 -> Data Store Write1/1
  CAN Unpack/3 -> Data Store Write2/1

== system ultra/RX/惯导/Subsystem3/Subsystem ==
  ID : Inport
  msg : Inport  Port=2
  Enable : EnablePort
  CAN Pack : canmsglib/CAN Pack  Commented=on  CANdbFile=D:\desktop\enable.dbc  MsgList=(none)  MsgName=AMK_ActualValue1  MsgIDType=Standard (11-bit identifier)  MsgIdentifier=643  MsgLength=8  Remote=off  ApplyMinMax=off  BusOutput=off  SignalInfo={'AMK_ActualVelocity','16','16','LE','signed','Standard','0','1','0','0','65535';'AMK_MagnetizingCurrent','48','16','LE','signed','Standard','0','1','0','0','65535';'AMK_TorqueCurrent','32','16','LE','signed','Standard','0','1','0','0','65535';'AMK_bDcOn1','12','1','LE','unsigned','Standard','0','1','0','0','1';'AMK_bDerating1','15','1','LE','unsigned','Standard','0','1','0','0','1';'AMK_bError1','9','1','LE','unsigned','Standard','0','1','0','0','1';'AMK_bInverterOn1','14','1','LE','unsigned','Standard','0','1','0','0','1';'AMK_bQuitDcOn1','11','1','LE','unsigned','Standard','0','1','0','0','1';'AMK_bQuitInverterOn1','13','1','LE','unsigned','Standard','0','1','0','0','1';'AMK_bReserve1','0','8','LE','unsigned','Standard','0','1','0','0','255';'AMK_bSystemReady1','8','1','LE','unsigned','Standard','0','1','0','0','1';'AMK_bWarn1','10','1','LE','unsigned','Standard','0','1','0','0','1'}
      settings: SourceProductBaseCode=ME,XP,VN  DataFormat=CANdb specified signals
  CAN Unpack : canmsglib/CAN Unpack  CANdbFile=C:\Users\Liu keliang\Desktop\HRT2023\HRT23赛季刘科良\CANdbc\homework1.dbc  MsgList=INS_Speed  MsgName=INS_Speed  MsgIDType=Standard (11-bit identifier)  MsgIdentifier=1285  MsgLength=7  SignalInfo={'INS_EastSpd','32','16','BE','unsigned','Standard','0','0.0030517','-100','-100','100';'INS_NorthSpd','16','16','BE','unsigned','Standard','0','0.0030517','-100','-100','100';'INS_ToGroundSpd','48','16','BE','unsigned','Standard','0','0.0030517','-100','-100','100'}  IDPort=off  TimestampPort=off  ErrorPort=off  RemotePort=off  LengthPort=off  StatusPort=off  ApplyMinMax=off
      settings: SourceProductBaseCode=ME,XP,VN  DataFormat=CANdb specified signals
  CANPackMessage : ec5744lib/RapidECU_U4B/04CANCommunication/CANPackMessage  Commented=on  datalength=8  sampletime=-1
      settings: SourceProductName=ECUCoder for MPC5744
  CANUnPackMessage : ec5744lib/RapidECU_U4B/04CANCommunication/CANUnPackMessage  datalength=7  canmessagetype=Standard(11-bit ID)  sampletime=-1
      settings: SourceProductName=ECUCoder for MPC5744
  Data Store Write : DataStoreWrite  DataStoreName=EAST_SPEED
  Data Store Write1 : DataStoreWrite  DataStoreName=NORTH_SPEED
  Data Store Write2 : DataStoreWrite  DataStoreName=TOGROUND_SPEED
  wires:
  msg/1 -> CANUnPackMessage/2
  CANUnPackMessage/1 -> CAN Unpack/1
  ID/1 -> CANUnPackMessage/1
  CANPackMessage/1 -> ?
  CAN Pack/1 -> CANPackMessage/1
  CAN Unpack/1 -> Data Store Write/1
  CAN Unpack/2 -> Data Store Write1/1
  CAN Unpack/3 -> Data Store Write2/1

== system ultra/RX/转向——receive1/Subsystem1/Subsystem ==
  ID : Inport
  msg : Inport  Port=2
  Enable : EnablePort
  CAN Pack : canmsglib/CAN Pack  Commented=on  CANdbFile=C:\Users\Liu keliang\Desktop\HRT2023\HRT23赛季刘科良\CANdbc\workstation.dbc  MsgList=(none)  MsgName=workstation  MsgIDType=Standard (11-bit identifier)  MsgIdentifier=32  MsgLength=5  Remote=off  ApplyMinMax=off  BusOutput=off  SignalInfo={'V','8','8','LE','unsigned','Standard','0','1','0','0','255';'V_Copy_1','16','8','LE','unsigned','Standard','0','1','0','0','255';'controlstart','4','1','LE','unsigned','Standard','0','1','0','-Inf','Inf';'status','0','4','LE','unsigned','Standard','0','1','0','0','15';'steering','24','8','LE','signed','Standard','0','1','0','-128','127';'steering_Copy_1','32','8','LE','signed','Standard','0','1','0','-128','127';'vfeedbackk','40','8','LE','unsigned','Standard','0','1','0','-Inf','Inf'}
      settings: SourceProductBaseCode=ME,XP,VN  DataFormat=CANdb specified signals
  CAN Unpack : canmsglib/CAN Unpack  CANdbFile=C:\Users\Liu keliang\Desktop\HRT2023\HRT23赛季刘科良\CANdbc\zhuanxiangbaocuo.dbc  MsgList=New_Message_1  MsgName=New_Message_1  MsgIDType=Standard (11-bit identifier)  MsgIdentifier=129  MsgLength=1  SignalInfo={'New_Signal_1','0','8','LE','signed','Standard','0','1','0','-Inf','Inf'}  IDPort=off  TimestampPort=off  ErrorPort=off  RemotePort=off  LengthPort=off  StatusPort=off  ApplyMinMax=off
      settings: SourceProductBaseCode=ME,XP,VN  DataFormat=CANdb specified signals
  CANPackMessage : ec5744lib/RapidECU_U4B/04CANCommunication/CANPackMessage  Commented=on  datalength=8  sampletime=-1
      settings: SourceProductName=ECUCoder for MPC5744
  CANUnPackMessage : ec5744lib/RapidECU_U4B/04CANCommunication/CANUnPackMessage  datalength=1  canmessagetype=Standard(11-bit ID)  sampletime=-1
      settings: SourceProductName=ECUCoder for MPC5744
  wires:
  msg/1 -> CANUnPackMessage/2
  CANUnPackMessage/1 -> CAN Unpack/1
  ID/1 -> CANUnPackMessage/1
  CANPackMessage/1 -> ?
  CAN Pack/1 -> CANPackMessage/1

== system ultra/RX/转向——receive1/Subsystem3/Subsystem ==
  ID : Inport
  msg : Inport  Port=2
  Enable : EnablePort
  CAN Pack : canmsglib/CAN Pack  Commented=on  CANdbFile=C:\Users\Liu keliang\Desktop\HRT2023\HRT23赛季刘科良\CANdbc\workstation.dbc  MsgList=(none)  MsgName=workstation  MsgIDType=Standard (11-bit identifier)  MsgIdentifier=32  MsgLength=5  Remote=off  ApplyMinMax=off  BusOutput=off  SignalInfo={'V','8','8','LE','unsigned','Standard','0','1','0','0','255';'V_Copy_1','16','8','LE','unsigned','Standard','0','1','0','0','255';'controlstart','4','1','LE','unsigned','Standard','0','1','0','-Inf','Inf';'status','0','4','LE','unsigned','Standard','0','1','0','0','15';'steering','24','8','LE','signed','Standard','0','1','0','-128','127';'steering_Copy_1','32','8','LE','signed','Standard','0','1','0','-128','127';'vfeedbackk','40','8','LE','unsigned','Standard','0','1','0','-Inf','Inf'}
      settings: SourceProductBaseCode=ME,XP,VN  DataFormat=CANdb specified signals
  CAN Unpack : canmsglib/CAN Unpack  CANdbFile=C:\Users\Liu keliang\Desktop\HRT2023\HRT23赛季刘科良\CANdbc\steering.dbc  MsgList=steeringfeedback  MsgName=steeringfeedback  MsgIDType=Standard (11-bit identifier)  MsgIdentifier=1153  MsgLength=6  SignalInfo={'konghzizi1','0','8','LE','signed','Standard','0','1','0','-Inf','Inf';'konghzizi1_Copy_1','8','8','LE','signed','Standard','0','1','0','-Inf','Inf';'targetposition','16','32','LE','signed','Standard','0','1','0','0','65535'}  IDPort=off  TimestampPort=off  ErrorPort=off  RemotePort=off  LengthPort=off  StatusPort=off  ApplyMinMax=off
      settings: SourceProductBaseCode=ME,XP,VN  DataFormat=CANdb specified signals
  CANPackMessage : ec5744lib/RapidECU_U4B/04CANCommunication/CANPackMessage  Commented=on  datalength=8  sampletime=-1
      settings: SourceProductName=ECUCoder for MPC5744
  CANUnPackMessage : ec5744lib/RapidECU_U4B/04CANCommunication/CANUnPackMessage  datalength=6  canmessagetype=Standard(11-bit ID)  sampletime=-1
      settings: SourceProductName=ECUCoder for MPC5744
  Data Store Write : DataStoreWrite  DataStoreName=steeringangle
  MATLAB Function : MATLAB Function  TreatAsAtomicUnit=on
  wires:
  msg/1 -> CANUnPackMessage/2
  CANUnPackMessage/1 -> CAN Unpack/1
  ID/1 -> CANUnPackMessage/1
  CANPackMessage/1 -> ?
  CAN Pack/1 -> CANPackMessage/1
  CAN Unpack/2 -> ?
  CAN Unpack/1 -> ?
  CAN Unpack/3 -> MATLAB Function/1(u)
  MATLAB Function/1(y) -> Data Store Write/1

== system ultra/RX/转向——receive编码器/Subsystem3/Subsystem ==
  ID : Inport
  msg : Inport  Port=2
  Enable : EnablePort
  CAN Pack : canmsglib/CAN Pack  Commented=on  CANdbFile=C:\Users\Liu keliang\Desktop\HRT2023\HRT23赛季刘科良\CANdbc\workstation.dbc  MsgList=(none)  MsgName=workstation  MsgIDType=Standard (11-bit identifier)  MsgIdentifier=32  MsgLength=5  Remote=off  ApplyMinMax=off  BusOutput=off  SignalInfo={'V','8','8','LE','unsigned','Standard','0','1','0','0','255';'V_Copy_1','16','8','LE','unsigned','Standard','0','1','0','0','255';'controlstart','4','1','LE','unsigned','Standard','0','1','0','-Inf','Inf';'status','0','4','LE','unsigned','Standard','0','1','0','0','15';'steering','24','8','LE','signed','Standard','0','1','0','-128','127';'steering_Copy_1','32','8','LE','signed','Standard','0','1','0','-128','127';'vfeedbackk','40','8','LE','unsigned','Standard','0','1','0','-Inf','Inf'}
      settings: SourceProductBaseCode=ME,XP,VN  DataFormat=CANdb specified signals
  CAN Unpack : canmsglib/CAN Unpack  CANdbFile=C:\Users\Liu keliang\Desktop\HRT2023\HRT23赛季刘科良\CANdbc\ZHUANJIAOBIANMAQI.dbc  MsgList=ZHUANJIAOBIIANMAQI  MsgName=ZHUANJIAOBIIANMAQI  MsgIDType=Standard (11-bit identifier)  MsgIdentifier=153  MsgLength=8  SignalInfo={'BUYONGGUAN','0','24','LE','signed','Standard','0','1','0','-Inf','Inf';'ZHUANJIAO','24','16','LE','unsigned','Standard','0','0.3516','0','-Inf','Inf'}  IDPort=off  TimestampPort=off  ErrorPort=off  RemotePort=off  LengthPort=off  StatusPort=off  ApplyMinMax=off
      settings: SourceProductBaseCode=ME,XP,VN  DataFormat=CANdb specified signals
  CANPackMessage : ec5744lib/RapidECU_U4B/04CANCommunication/CANPackMessage  Commented=on  datalength=8  sampletime=-1
      settings: SourceProductName=ECUCoder for MPC5744
  CANUnPackMessage : ec5744lib/RapidECU_U4B/04CANCommunication/CANUnPackMessage  datalength=8  canmessagetype=Standard(11-bit ID)  sampletime=-1
      settings: SourceProductName=ECUCoder for MPC5744
  Data Store Write : DataStoreWrite  DataStoreName=zhuanjiaobianmaqi
  Data Store Write1 : DataStoreWrite  DataStoreName=zhuanjiaoweigeniubi
  MATLAB Function : MATLAB Function  TreatAsAtomicUnit=on
  wires:
  msg/1 -> CANUnPackMessage/2
  CANUnPackMessage/1 -> CAN Unpack/1
  ID/1 -> CANUnPackMessage/1
  CANPackMessage/1 -> ?
  CAN Pack/1 -> CANPackMessage/1
  CAN Unpack/2 -> Data Store Write1/1, MATLAB Function/1(u)
  MATLAB Function/1(y) -> Data Store Write/1
